simulink model "MRAC_NL"  (R2022b)
settings: Solver=VariableStepAuto  StartTime=0.0  StopTime=200  RelTol=1e-3
values from neighbouring files (symbols this model uses):
  d1 = 0.13075    [TF.mat]
  d2 = 0.05075    [TF.mat]
  DZ = 3    [TF.mat]
  gamma_r = 0.3    [MRAC.mat]
  Gamma_x = 7    [MRAC.mat]
  I = 0.00015    [TF.mat]
  km = 0.001118    [TF.mat]
  MAX_PWM = 80    [TF.mat]
  miu = 0.0005001    [TF.mat]
  wb = 0.105948    [TF.mat]
  wcp = 0.014145    [TF.mat]
  wm = 0.030411    [TF.mat]
undefined symbols (not defined in the file or in its folder): GMRAC, GRM, Gss, Observer, Pbarra
settings Model: Creator=andre  LastModifiedBy=felip
settings DebuggingCC: UnconnectedInputMsg=warning  UnconnectedOutputMsg=warning  UnconnectedLineMsg=warning  SFMachineParentedDataDiag=warning
settings ModelReferenceCC: EnableRefExpFcnMdlSchedulingChecks=on
settings RTWCC: DLArmComputeVersion=19.05

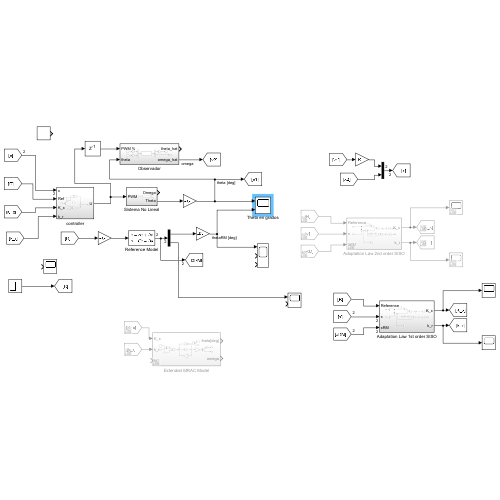
[thumbnail: Simulink's stored preview of the top-level diagram]
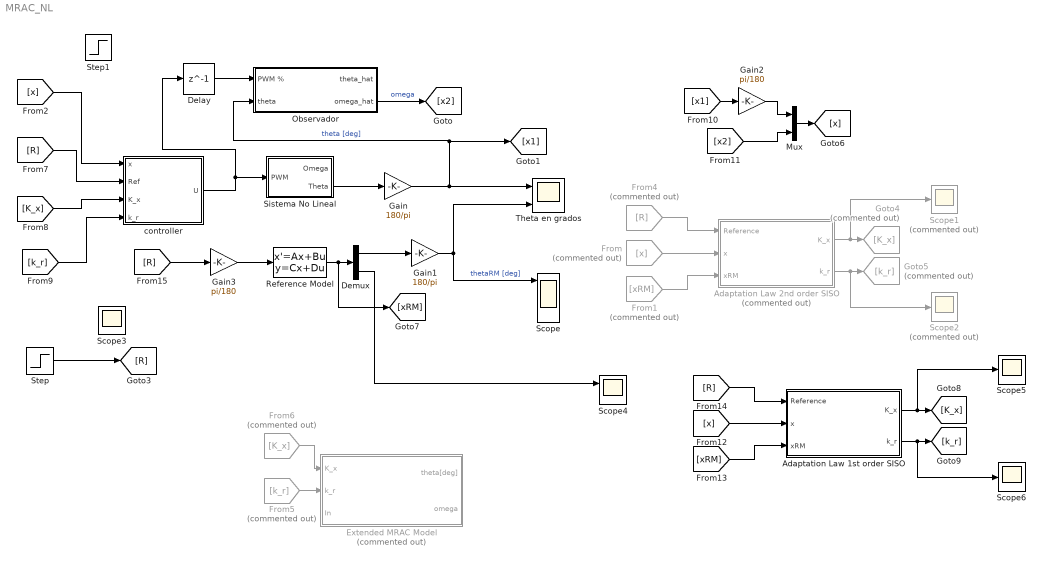
== system MRAC_NL ==
  Adaptation Law 1st order SISO : Subsystem
  Adaptation Law 2nd order SISO : Subsystem  Commented=on
  Delay : Delay  DelayLength=1
  Demux : Demux  Outputs=2
  Extended MRAC Model : Subsystem  Commented=on
  From : From  Commented=on  GotoTag=x
  From1 : From  Commented=on  GotoTag=xRM
  From4 : From  Commented=on  GotoTag=R
  From5 : From  Commented=on  GotoTag=k_r
  From6 : From  Commented=on  GotoTag=K_x
  Gain : Gain  Gain=180/pi
  Gain1 : Gain  Gain=180/pi
  Gain2 : Gain  Gain=pi/180
  Gain3 : Gain  Gain=pi/180
  Goto4 : Goto  Commented=on  GotoTag=K_x
  Goto5 : Goto  Commented=on  GotoTag=k_r
  Mux : Mux  Inputs=2
  Observador : Subsystem
  Reference Model : StateSpace  A=GRM.A  B=GRM.B  C=GRM.C  D=GRM.D  InitialCondition=0
  Scope : Scope  NumInputPorts=3
  Scope1 : Scope  Commented=on
  Scope2 : Scope  Commented=on
  Scope3 : Scope
  Scope4 : Scope  NumInputPorts=2
  Scope5 : Scope
  Scope6 : Scope
  Sistema No Lineal : Subsystem
  Step : Step  Time=0  After=20  SampleTime=0
  Step1 : Step  SampleTime=0
  Theta en grados : Scope  NumInputPorts=2
  controller : Subsystem
  wires:
  Sistema No Lineal/2(Theta) -> Gain/1
  Gain/1 -> [x1], Observador/2(theta), Theta en grados/1  "theta [deg]"
  Observador/2(omega_hat) -> [x2]  "omega"
  Reference Model/1 -> [xRM], Demux/1
  From4/1 -> Adaptation Law 2nd order SISO/1(Reference)
  Adaptation Law 2nd order SISO/1(K_x) -> Scope1/1, Goto4/1
  Adaptation Law 2nd order SISO/2(k_r) -> Scope2/1, Goto5/1
  [x] -> controller/1(x)
  [R] -> controller/2(Ref)
  Step/1 -> [R]
  [K_x] -> controller/3(K_x)
  [k_r] -> controller/4(k_r)
  [x1] -> Gain2/1
  Gain2/1 -> Mux/1
  [x2] -> Mux/2
  Mux/1 -> [x]
  From/1 -> Adaptation Law 2nd order SISO/2(x)
  From1/1 -> Adaptation Law 2nd order SISO/3(xRM)
  From5/1 -> Extended MRAC Model/2(k_r)
  From6/1 -> Extended MRAC Model/1(K_x)
  Demux/2 -> Scope4/1
  [x] -> Adaptation Law 1st order SISO/2(x)
  [xRM] -> Adaptation Law 1st order SISO/3(xRM)
  Adaptation Law 1st order SISO/2(k_r) -> Scope6/1, [k_r]
  Adaptation Law 1st order SISO/1(K_x) -> Scope5/1, [K_x]
  [R] -> Adaptation Law 1st order SISO/1(Reference)
  Delay/1 -> Observador/1(PWM %)
  Demux/1 -> Gain1/1
  Gain1/1 -> Theta en grados/2, Scope/1  "thetaRM [deg]"
  Gain3/1 -> Reference Model/1
  [R] -> Gain3/1
  controller/1(U) -> Delay/1, Sistema No Lineal/1(PWM)

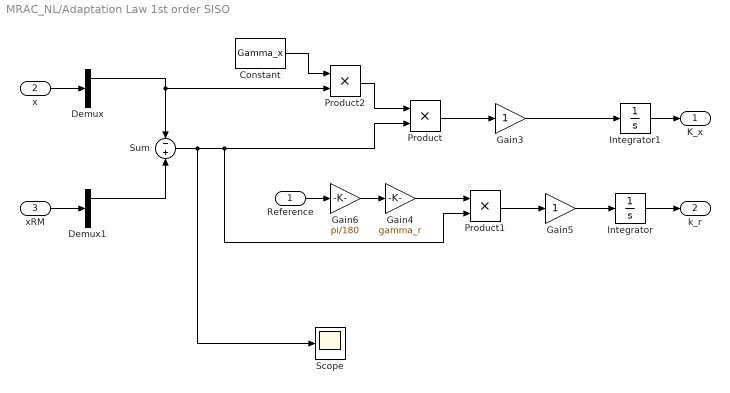
== system MRAC_NL/Adaptation Law 1st order SISO ==
  Reference : Inport
  x : Inport  Port=2
  xRM : Inport  Port=3
  Constant : Constant  Value=Gamma_x
  Demux : Demux  Outputs=2
  Demux1 : Demux  Outputs=2
  Gain3 : Gain
  Gain4 : Gain  Gain=gamma_r
  Gain5 : Gain
  Gain6 : Gain  Gain=pi/180
  Integrator : Integrator
  Integrator1 : Integrator
  Product : Product
  Product1 : Product
  Product2 : Product
  Scope : Scope
  Sum : Sum  Inputs=-+
  K_x : Outport
  k_r : Outport  Port=2
  wires:
  Product/1 -> Gain3/1
  Gain5/1 -> Integrator/1
  Gain4/1 -> Product1/1
  Product1/1 -> Gain5/1
  Reference/1 -> Gain6/1
  Sum/1 -> Product1/2, Product/2, Scope/1
  Gain6/1 -> Gain4/1
  Product2/1 -> Product/1
  Constant/1 -> Product2/1
  Integrator/1 -> k_r/1
  Integrator1/1 -> K_x/1
  x/1 -> Demux/1
  Demux/1 -> Product2/2, Sum/1
  xRM/1 -> Demux1/1
  Demux1/1 -> Sum/2
  Gain3/1 -> Integrator1/1

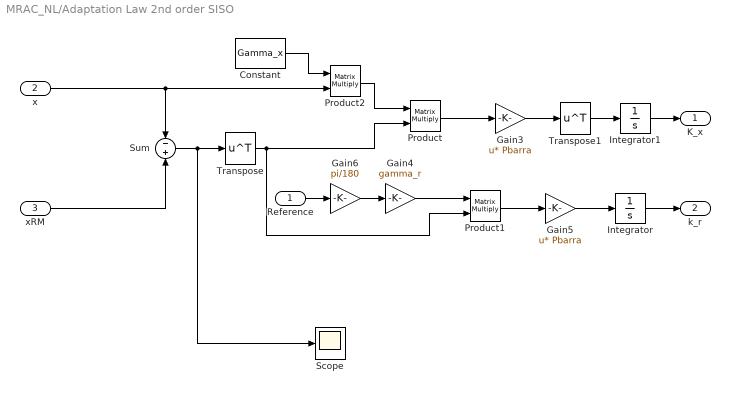
== system MRAC_NL/Adaptation Law 2nd order SISO ==
  Reference : Inport
  x : Inport  Port=2
  xRM : Inport  Port=3
  Constant : Constant  Value=Gamma_x
  Gain3 : Gain  Gain=Pbarra  Multiplication=Matrix(u*K)
  Gain4 : Gain  Gain=gamma_r
  Gain5 : Gain  Gain=Pbarra  Multiplication=Matrix(u*K)
  Gain6 : Gain  Gain=pi/180
  Integrator : Integrator
  Integrator1 : Integrator
  Product : Product  Multiplication=Matrix(*)
  Product1 : Product  Multiplication=Matrix(*)
  Product2 : Product  Multiplication=Matrix(*)
  Scope : Scope
  Sum : Sum  Inputs=-+
  Transpose : Math  Operator=transpose
  Transpose1 : Math  Operator=transpose
  K_x : Outport
  k_r : Outport  Port=2
  wires:
  Sum/1 -> Scope/1, Transpose/1
  Product/1 -> Gain3/1
  Gain5/1 -> Integrator/1
  Gain4/1 -> Product1/1
  Product1/1 -> Gain5/1
  Reference/1 -> Gain6/1
  Transpose/1 -> Product/2, Product1/2
  Gain6/1 -> Gain4/1
  Product2/1 -> Product/1
  Constant/1 -> Product2/1
  Gain3/1 -> Transpose1/1
  Transpose1/1 -> Integrator1/1
  xRM/1 -> Sum/2
  x/1 -> Sum/1, Product2/2
  Integrator/1 -> k_r/1
  Integrator1/1 -> K_x/1

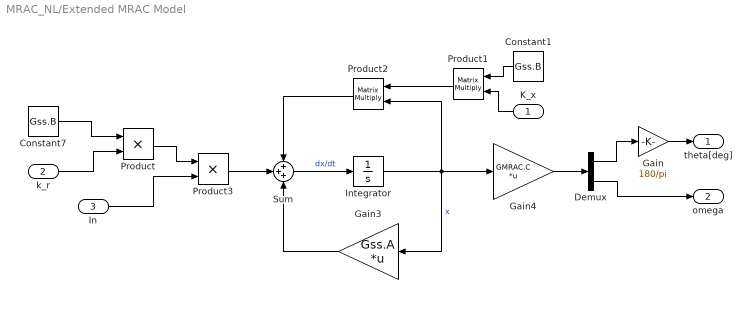
== system MRAC_NL/Extended MRAC Model ==
  K_x : Inport
  k_r : Inport  Port=2
  In : Inport  Port=3
  Constant1 : Constant  Value=Gss.B
  Constant7 : Constant  Value=Gss.B
  Demux : Demux  Outputs=2
  Gain : Gain  Gain=180/pi
  Gain3 : Gain  Gain=Gss.A  Multiplication=Matrix(K*u)
  Gain4 : Gain  Gain=GMRAC.C  Multiplication=Matrix(K*u)
  Integrator : Integrator
  Product : Product
  Product1 : Product  Multiplication=Matrix(*)
  Product2 : Product  Multiplication=Matrix(*)
  Product3 : Product
  Sum : Sum  Inputs=+++
  theta[deg] : Outport
  omega : Outport  Port=2
  wires:
  Integrator/1 -> Product2/2, Gain4/1, Gain3/1  "x"
  Constant7/1 -> Product/1
  Sum/1 -> Integrator/1  "dx/dt"
  k_r/1 -> Product/2
  Constant1/1 -> Product1/1
  K_x/1 -> Product1/2
  Gain3/1 -> Sum/3
  Product2/1 -> Sum/1
  Product1/1 -> Product2/1
  Gain4/1 -> Demux/1
  Product3/1 -> Sum/2
  Product/1 -> Product3/1
  In/1 -> Product3/2
  Demux/1 -> Gain/1
  Gain/1 -> theta[deg]/1
  Demux/2 -> omega/1

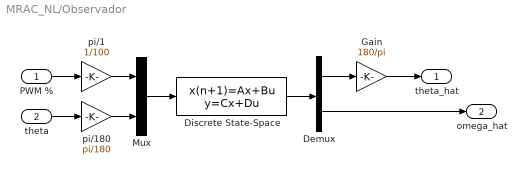
== system MRAC_NL/Observador ==
  PWM % : Inport
  theta : Inport  Port=2
  Demux : Demux  Outputs=2
  Discrete State-Space : DiscreteStateSpace  A=Observer.A  B=Observer.B  C=Observer.C  D=Observer.D  SampleTime=-1
  Gain : Gain  Gain=180/pi
  Mux : Mux  Inputs=2
  pi/1 : Gain  Gain=1/100
  pi/180 : Gain  Gain=pi/180
  theta_hat : Outport
  omega_hat : Outport  Port=2  Unit=rad/sec
  wires:
  Mux/1 -> Discrete State-Space/1
  theta/1 -> pi/180/1
  Discrete State-Space/1 -> Demux/1
  pi/180/1 -> Mux/2
  PWM %/1 -> pi/1/1
  pi/1/1 -> Mux/1
  Gain/1 -> theta_hat/1
  Demux/1 -> Gain/1
  Demux/2 -> omega_hat/1

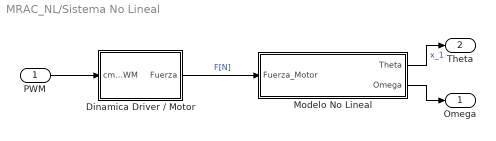
== system MRAC_NL/Sistema No Lineal ==
  PWM : Inport
  Dinamica Driver / Motor : Subsystem
  Modelo No Lineal : Subsystem
  Omega : Outport
  Theta : Outport  Port=2
  wires:
  PWM/1 -> Dinamica Driver / Motor/1(cmd_PWM)
  Dinamica Driver / Motor/1(Fuerza) -> Modelo No Lineal/1(Fuerza_Motor)  "F[N]"
  Modelo No Lineal/1(Theta) -> Theta/1  "x_1"
  Modelo No Lineal/2(Omega) -> Omega/1

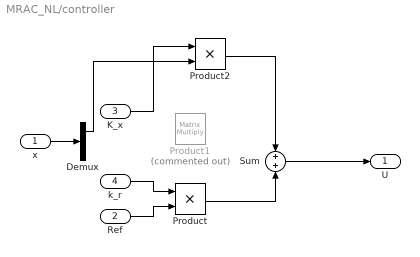
== system MRAC_NL/controller ==
  x : Inport
  Ref : Inport  Port=2
  K_x : Inport  Port=3
  k_r : Inport  Port=4
  Demux : Demux  Outputs=2
  Product : Product
  Product1 : Product  Commented=on  Multiplication=Matrix(*)
  Product2 : Product
  Sum : Sum
  U : Outport
  wires:
  Ref/1 -> Product/2
  Product/1 -> Sum/2
  k_r/1 -> Product/1
  K_x/1 -> Product2/1
  Sum/1 -> U/1
  x/1 -> Demux/1
  Demux/1 -> Product2/2
  Product2/1 -> Sum/1

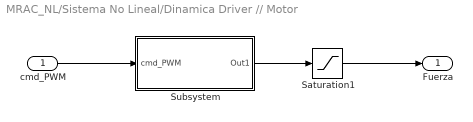
== system MRAC_NL/Sistema No Lineal/Dinamica Driver // Motor ==
  cmd_PWM : Inport
  Saturation1 : Saturate  UpperLimit=MAX_PWM  ZeroCross=off
  Subsystem : Subsystem
  Fuerza : Outport
  wires:
  Saturation1/1 -> Fuerza/1
  cmd_PWM/1 -> Subsystem/1(cmd_PWM)
  Subsystem/1(Out1) -> Saturation1/1

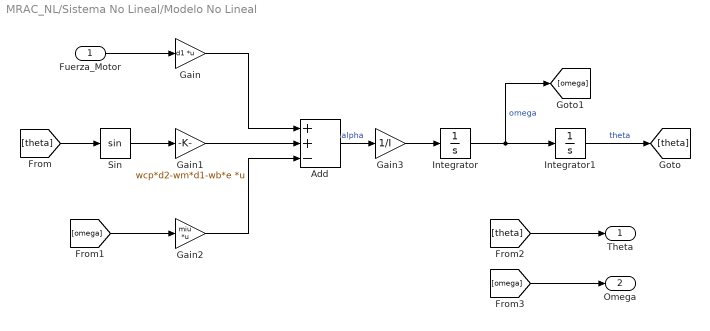
== system MRAC_NL/Sistema No Lineal/Modelo No Lineal ==
  Fuerza_Motor : Inport
  Add : Sum  Inputs=++-
  Gain : Gain  Gain=d1  Multiplication=Matrix(K*u)
  Gain1 : Gain  Gain=wcp*d2-wm*d1-wb*e  Multiplication=Matrix(K*u)
  Gain2 : Gain  Gain=miu  Multiplication=Matrix(K*u)
  Gain3 : Gain  Gain=1/I
  Integrator : Integrator  ZeroCross=off
  Integrator1 : Integrator  ZeroCross=off
  Sin : Trigonometry
  Theta : Outport
  Omega : Outport  Port=2
  wires:
  [omega] -> Omega/1
  Gain1/1 -> Add/2
  Integrator/1 -> [omega], Integrator1/1  "omega"
  Fuerza_Motor/1 -> Gain/1
  Integrator1/1 -> [theta]  "theta"
  Gain2/1 -> Add/3
  Gain/1 -> Add/1
  Add/1 -> Gain3/1  "alpha"
  [theta] -> Sin/1
  [omega] -> Gain2/1
  [theta] -> Theta/1
  Sin/1 -> Gain1/1
  Gain3/1 -> Integrator/1

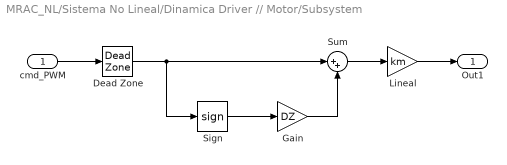
== system MRAC_NL/Sistema No Lineal/Dinamica Driver // Motor/Subsystem ==
  cmd_PWM : Inport
  Dead Zone : DeadZone  LowerValue=-DZ  UpperValue=DZ  ZeroCross=off
  Gain : Gain  Gain=DZ
  Lineal : Gain  Gain=km
  Sign : Signum  ZeroCross=off
  Sum : Sum  Inputs=|++
  Out1 : Outport
  wires:
  cmd_PWM/1 -> Dead Zone/1
  Dead Zone/1 -> Sum/1, Sign/1
  Sum/1 -> Lineal/1
  Sign/1 -> Gain/1
  Gain/1 -> Sum/2
  Lineal/1 -> Out1/1
